simulink model "sizing_test"  (R2020b)
settings: Solver=FixedStepAuto  StartTime=0.0  StopTime=inf  RelTol=1e-3  EnableMultiTasking=on
settings Model: SILPILModeSetting=veronly  ExtModeTrigDuration=2  Creator=tcbir  LastModifiedBy=tcbir
settings DataIOCC: SaveOutput=off  SignalLogging=off  DSMLogging=off  SaveTime=off  ReturnWorkspaceOutputs=off
settings OptimizationCC: DefaultUnderspecifiedDataType=single  EnhancedBackFolding=on  PassReuseOutputArgsAs=Individual arguments  ZeroExternalMemoryAtStartup=off  ZeroInternalMemoryAtStartup=off  MaxStackSize=64  OptimizeBlockOrder=speed  DifferentSizesBufferReuse=on  OptimizationCustomize=off  EfficientTunableParamExpr=on
settings DebuggingCC: ParameterTunabilityLossMsg=error
settings HardwareCC: ProdBitPerInt=16  ProdBitPerPointer=16  ProdBitPerSizeT=16  ProdBitPerPtrDiffT=16  ProdLargestAtomicFloat=None  ProdWordSize=8  ProdHWDeviceType=Atmel->AVR  UseEmbeddedCoderFeatures=off  UseSimulinkCoderFeatures=off
settings SFSimCC: MATLABDynamicMemAlloc=off
settings RTWCC: Description=Embedded Coder  SystemTargetFile=ert.tlc  HardwareBoard=Arduino Mega 2560  TemplateMakefile=ert_default_tmf  Toolchain=Arduino AVR  BuildConfiguration=Faster Runs
settings CodeAppCC: ForceParamTrailComments=on  IgnoreCustomStorageClasses=off  OperatorAnnotations=on  SimulinkDataObjDesc=on  SFDataObjDesc=on  InsertBlockDesc=on
settings ERTTargetCC: SupportContinuousTime=on  SupportNonInlinedSFcns=on  SupportVariableSizeSignals=on  ExtModeStaticAllocSize=2048

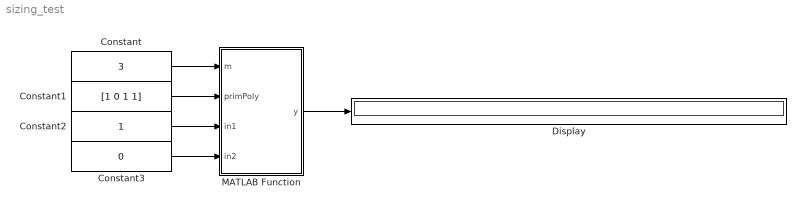
== system sizing_test ==
  Constant : Constant  Value=3
  Constant1 : Constant  Value=[1 0 1 1]
  Constant2 : Constant
  Constant3 : Constant  Value=0
  Display : Display
  MATLAB Function : MATLAB Function  TreatAsAtomicUnit=on
  wires:
  MATLAB Function/1(y) -> Display/1
  Constant/1 -> MATLAB Function/1(m)
  Constant3/1 -> MATLAB Function/4(in2)
  Constant2/1 -> MATLAB Function/3(in1)
  Constant1/1 -> MATLAB Function/2(primPoly)

== matlab function sizing_test/MATLAB Function ==
  data: m input; y output; primPoly input; in1 input; in2 input

function y = fcn(m, primPoly, in1, in2) %dummy_vector is only used to define the size of the output

    gf = GenerateGF2m(int8(m), int8(primPoly));
    y = AddGF2m(int8(in1), int8(in2), int8(gf), int8(m));

end


function gf  = GenerateGF2m(m, primPoly) %primPoly in power notation, highest order on left

    %m = 3;
    % hard coded size of retrun matrices and gf mtrix because simulink
    % whines about variable output size. Havent figured out how to fix it
    % ask laberge
    gf = int8(zeros(8, m)); %there are 2^m field elements
    %field_elements = zeros(8, int8(m)); %there are 2^m field elements

    numShifts = int8((2^m) - 1);
    s_reg = int8(zeros(1,int8(m)));
    s_reg(end) = int8(1); %rightmost element of init shr is 1
    gf(1, :) = int8(0);%write the contents of the init shift register to the matrix of gf elements
    gf(2, :) = int8(s_reg);
    for i = 2:numShifts %number of shifts corresponds to power of primitive element
        carryOut = int8(s_reg(1));%save the value to be wrapped
        for i0 = 1:numel(s_reg)-1
            if primPoly(i0 + 1) == 1
                s_reg(i0) = int8(xor(carryOut, s_reg(i0 + 1)));
            else
                s_reg(i0) = int8(s_reg(i0 + 1));
            end
        end
        s_reg(end) = int8(carryOut);
        gf(i+1,:) = int8(s_reg); %add the newly shifted register to the gf matrix
    end
end

function [sum] = AddGF2m(in1, in2, gf_matrix, m)
    %m = numel(gf_matrix(1,:));
    %convert power notation to rectangular
    if in1 == -1
        sum = int8(in2);
    elseif in2 == -1
        sum = int8(in1);
    elseif in1 == in2
        sum = int8(-1); %changed
    else
        % had to put this sum = 0 here bacsue simulink whines about sum not
        % begin initialized in some decision trees
        sum = int8(0);
        gfIndx = int8(in1 + 2); %account for inf and indexing
        r_in1 = int8(gf_matrix(gfIndx, :));

        if in2 == -1
            r_in2 = int8(zeros(1, m));
        else
            gfIndx = in2 + 2; %account for inf and indexing
            r_in2 = int8(gf_matrix(gfIndx, :));
        end

        xor_res = int8(xor(r_in1, r_in2)); %xor the rectangular coordinates
        [rows, ~] = size(gf_matrix);

        for i = 1:rows %check each row of GF for matches
            if xor_res(1,:) == int8(gf_matrix(i,:))
                if i == 1
                    sum = int8(-1);
                else
                    sum = int8(i - 2);%reverse indexing from above
                end
                break;
            end
        end
    end 
end
